simulink model "EKF_04_2014"  (R2015a)
settings: Solver=ode45  StartTime=0.0  StopTime=200  RelTol=1e-3
model workspace: external: MATLAB File Init_Model_02_Simulink.m (data not in the file)
values from neighbouring files (symbols this model uses):
  Cov_nu = [0.005 0 0 0 ... (first row only)    [InitOOSM.m]    (also in InitSIL.m; Init_Model_02_Simulink.m; Init_Model_02_Simulink_SIL1.m)
  Cov_r = [0.003 0 0 ... (first row only)    [InitOOSM.m]    (also in InitSIL.m; Init_Model_02_Simulink.m; Init_Model_02_Simulink_SIL1.m)
  e_force_x = 0    [InitOOSM.m]    (also in InitSIL.m; Init_Model_02_Simulink.m; Init_Model_02_Simulink_SIL1.m)
  e_force_y = 0    [InitOOSM.m]    (also in InitSIL.m; Init_Model_02_Simulink.m; Init_Model_02_Simulink_SIL1.m)
  e_force_z = 0    [InitOOSM.m]    (also in InitSIL.m; Init_Model_02_Simulink.m; Init_Model_02_Simulink_SIL1.m)
  ita = [0.5;0.5;0.5;0.5]    [InitOOSM.m]    (also in InitSIL.m; Init_Model_02_Simulink.m = [0.12; 0.05; -0.15; 0.98]; Init_Model_02_Simulink_SIL1.m)
  n = 0.00    (= 0)    [InitOOSM.m]    (also in InitSIL.m; Init_Model_02_Simulink.m = 0.0012; Init_Model_02_Simulink_SIL1.m)
  P_d = Simulink.Signal    [InitOOSM.m]    (also in InitSIL.m; Init_Model_02_Simulink.m; Init_Model_02_Simulink_SIL1.m)
  P_k = Simulink.Signal    [InitOOSM.m]    (also in InitSIL.m; Init_Model_02_Simulink.m; Init_Model_02_Simulink_SIL1.m)
  p_x = 0.75    [InitOOSM.m]    (also in InitSIL.m; Init_Model_02_Simulink.m; Init_Model_02_Simulink_SIL1.m)
  p_y = 0.125    [InitOOSM.m]    (also in InitSIL.m; Init_Model_02_Simulink.m; Init_Model_02_Simulink_SIL1.m)
  p_z = -0.8    [InitOOSM.m]    (also in InitSIL.m; Init_Model_02_Simulink.m; Init_Model_02_Simulink_SIL1.m)
  parameter_gravitation = 3.986005E+14    (= 398600500000000)    [InitOOSM.m]    (also in InitSIL.m; Init_Model_02_Simulink.m; Init_Model_02_Simulink_SIL1.m)
  rho = [0.04;0;0.3]    [InitOOSM.m]    (also in InitSIL.m; Init_Model_02_Simulink.m = [0.2; 0.1; 0.05]; Init_Model_02_Simulink_SIL1.m)
  rho_c = [-0.00017;   -0.9780;   -0.1854]    [InitOOSM.m]    (also in InitSIL.m = [0.00036;   -0.9865;   -0.1854]; Init_Model_02_Simulink.m = [0; 0; 0.9]; Init_Model_02_Simulink_SIL1.m = [0.00036;   -0.9865;   -0.1854])
  sig_f = 2E-6    (= 2e-06)    [InitOOSM.m]    (also in InitSIL.m; Init_Model_02_Simulink.m; Init_Model_02_Simulink_SIL1.m)
  sig_tau = 2.5E-5    (= 2.5e-05)    [InitOOSM.m]    (also in InitSIL.m; Init_Model_02_Simulink.m; Init_Model_02_Simulink_SIL1.m)
  t_delta = 0.2    [InitOOSM.m]    (also in InitSIL.m; Init_Model_02_Simulink.m = 0.1; Init_Model_02_Simulink_SIL1.m)
  t_Kalman = 0.01    [InitOOSM.m]    (also in InitSIL.m; Init_Model_02_Simulink.m; Init_Model_02_Simulink_SIL1.m)
  t_Sim = 0.001    [InitOOSM.m]    (also in InitSIL.m; Init_Model_02_Simulink.m; Init_Model_02_Simulink_SIL1.m)
  tau_1 = 0    [InitOOSM.m]    (also in InitSIL.m; Init_Model_02_Simulink.m; Init_Model_02_Simulink_SIL1.m)
  tau_2 = 0    [InitOOSM.m]    (also in InitSIL.m; Init_Model_02_Simulink.m; Init_Model_02_Simulink_SIL1.m)
  tau_3 = 0    [InitOOSM.m]    (also in InitSIL.m; Init_Model_02_Simulink.m; Init_Model_02_Simulink_SIL1.m)
  U_n_d = Simulink.Signal    [InitOOSM.m]    (also in InitSIL.m; Init_Model_02_Simulink.m; Init_Model_02_Simulink_SIL1.m)
  W_0 = [1 0 0 0 0 0 ... (first row only)    [InitOOSM.m]    (also in InitSIL.m; Init_Model_02_Simulink.m; Init_Model_02_Simulink_SIL1.m)
  X_a_0 = [0; 0; 0; 1; 0; 0; 0; 0; 0; 0; 0; 0; 0;0;0;0;0;0;0;1]    [InitOOSM.m]    (also in InitSIL.m = [0; 0; 0; 1; 0; 0; 0; 0; 0; 0; 0; 0; 0]; Init_Model_02_Simulink.m = [0; 0; 0; 1; 0; 0; 0; 0; 0; 0; 0; 0; 0]; Init_Model_02_Simulink_SIL1.m = [0;0;0.707;0.707;0.2;-0.02;0.0001;0.02;-1.80;0.50;-0.05;0.00)
  x_d = Simulink.Signal    [InitOOSM.m]    (also in InitSIL.m; Init_Model_02_Simulink.m; Init_Model_02_Simulink_SIL1.m)
  x_k = Simulink.Signal    [InitOOSM.m]    (also in InitSIL.m; Init_Model_02_Simulink.m; Init_Model_02_Simulink_SIL1.m)
undefined symbols (not defined in the file or in its folder): des, gcbh
libraries: simulink x8, dspmtrx3 x2, visionstatistics x1
(part 1 of 5)
settings Model: PauseTimes=0.19  NumberOfSteps=10  SnapshotBufferSize=1  CovSFcnEnable=off  Creator=Iseberg  LastModifiedBy=Ana
settings DebuggingCC: SolverPrmCheckMsg=warning

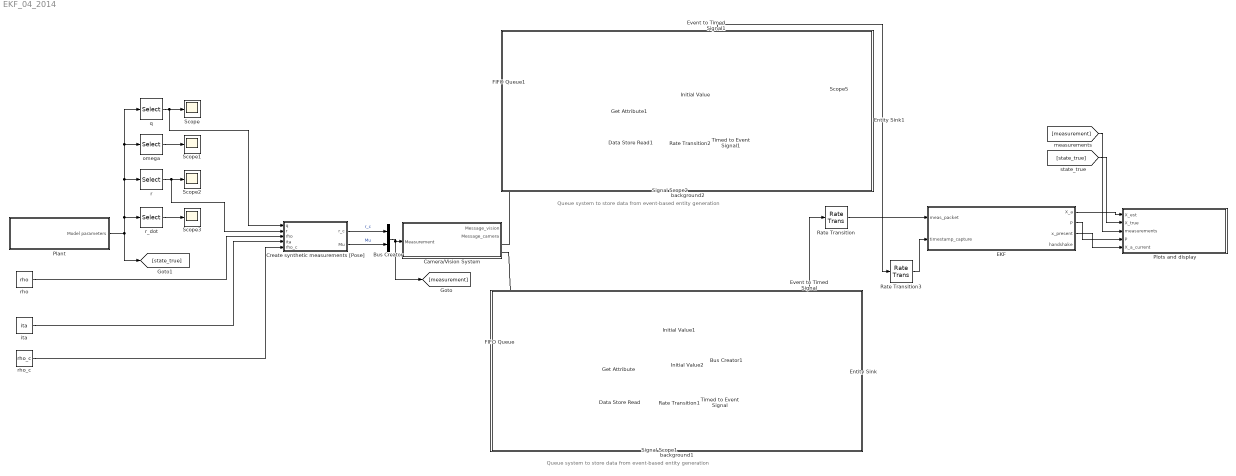
== system EKF_04_2014 ==
  note: Queue system to store data from event-based entity generation
  note: Queue system to store data from event-based entity generation
  Bus Creator : BusCreator  Inputs=2
  Bus Creator1 : BusCreator  Inputs=3
  Camera/Vision System : Subsystem
  Create synthetic measurements [Pose] : Subsystem  TreatAsAtomicUnit=on
  Data Store Read : DataStoreRead  DataStoreName=flag_queue
  Data Store Read1 : DataStoreRead  DataStoreName=flag_queue
  EKF : Subsystem  TreatAsAtomicUnit=on  SystemSampleTime=t_Kalman
  Entity Sink : EntitySink
  Entity Sink1 : EntitySink
  Event to Timed Signal : EventToTimedSignal
  Event to Timed Signal1 : EventToTimedSignal
  FIFO Queue : FIFOQueue  StatNumberInBlock=on
      settings: OutputPortMap=o1
  FIFO Queue1 : FIFOQueue  StatNumberInBlock=on
      settings: OutputPortMap=o1
  Get Attribute : GetAttribute  AttributeName=meas_vector|timestamp_capture|timestamp_processed  AttributeMissing=Error|Error|Error  AttributeDefaultValue=1|1|1  AttributeTreatAsVector=1|1|1  AttributeSendTiming=After entity departure|After entity departure|After entity departure  EvaluatedDefaultAttributeValue={ [];[];[]}
      settings: OutputPortMap=o1,o2,o3
  Get Attribute1 : GetAttribute  AttributeName=timestamp_capture  EvaluatedDefaultAttributeValue={ []}
      settings: OutputPortMap=o1
  Initial Value : InitialValue  InitialValue=-1
  Initial Value1 : InitialValue  InitialValue=-1
  Initial Value2 : InitialValue  InitialValue=-1
  Plant : Subsystem
  Plots and display : Subsystem
  Rate Transition{,1..3} (4 alike) : RateTransition  OutPortSampleTime=t_Kalman
  Scope{,1..3,5} (5 alike) : Scope
      Scope settings: ShowLegends=on  YMin=-1  YMax=1  MaxDataPoints=100000
      Scope1 settings: ShowLegends=on  TimeRange=40
      Scope2 settings: ShowLegends=on  SaveName=ScopeData2
      Scope3 settings: ShowLegends=on  SaveName=ScopeData3
      Scope5 settings: SaveName=ScopeData12
  Signal Scope1 : SignalScope  LoadFcn=des.scope.CallbackSupport('seLoadFcn',gcbh)  StartFcn=des.scope.CallbackSupport('seStartFcn',gcbh)  StopFcn=des.scope.CallbackSupport('seStopFcn',gcbh)
      settings: CopyFcn=des.scope.CallbackSupport('seCopyFcn',gcbh)  DeleteFcn=des.scope.CallbackSupport('seDeleteFcn',gcbh)  PreSaveFcn=des.scope.CallbackSupport('sePreSaveFcn',gcbh)  NameChangeFcn=des.scope.CallbackSupport('seNameChangeFcn',gcbh)  OpenFcn=des.scope.CallbackSupport('seOpenFcn',gcbh)
  Signal Scope2 : SignalScope  LoadFcn=des.scope.CallbackSupport('seLoadFcn',gcbh)  StartFcn=des.scope.CallbackSupport('seStartFcn',gcbh)  StopFcn=des.scope.CallbackSupport('seStopFcn',gcbh)
      settings: CopyFcn=des.scope.CallbackSupport('seCopyFcn',gcbh)  DeleteFcn=des.scope.CallbackSupport('seDeleteFcn',gcbh)  PreSaveFcn=des.scope.CallbackSupport('sePreSaveFcn',gcbh)  NameChangeFcn=des.scope.CallbackSupport('seNameChangeFcn',gcbh)  OpenFcn=des.scope.CallbackSupport('seOpenFcn',gcbh)
  Timed to Event Signal : TimedToEventSignal
  Timed to Event Signal1 : TimedToEventSignal
  background1 : Subsystem
      mask Display: disp('')
  background2 : Subsystem
      mask Display: disp('')
  ita : Constant  Value=ita
  omega : Selector  NumberOfDimensions=2  InputPortWidth=3  IndexOptions=Index vector (dialog),Index vector (dialog)  Indices=[5 6 7],1  OutputSizes=1,1
  q : Selector  NumberOfDimensions=2  InputPortWidth=3  IndexOptions=Index vector (dialog),Index vector (dialog)  Indices=[1 2 3 4],1  OutputSizes=1,1
  r : Selector  NumberOfDimensions=2  InputPortWidth=3  IndexOptions=Index vector (dialog),Index vector (dialog)  Indices=[8 9 10],1  OutputSizes=1,1
  r_dot : Selector  NumberOfDimensions=2  InputPortWidth=3  IndexOptions=Index vector (dialog),Index vector (dialog)  Indices=[11 12 13],1  OutputSizes=1,1
  "rho " : Constant  Value=rho
  rho_c : Constant  Value=rho_c
  wires:
  omega/1 -> Scope1/1
  r_dot/1 -> Scope3/1
  Plant/1(Model parameters) -> [state_true], omega/1, q/1, r/1, r_dot/1
  q/1 -> Create synthetic measurements [Pose]/1(q), Scope/1
  r/1 -> Create synthetic measurements [Pose]/2(r), Scope2/1
  "rho "/1 -> Create synthetic measurements [Pose]/3(rho)
  ita/1 -> Create synthetic measurements [Pose]/4(ita)
  rho_c/1 -> Create synthetic measurements [Pose]/5("rho_c ")
  Create synthetic measurements [Pose]/1(r_c) -> Bus Creator/1  "r_c"
  Create synthetic measurements [Pose]/2(Mu) -> Bus Creator/2  "Mu"
  Bus Creator/1 -> [measurement], Camera/Vision System/1(Measurement)
  Bus Creator1/1 -> Event to Timed Signal/1
  FIFO Queue/1 -> Signal Scope1/1
  Get Attribute/2 -> Initial Value1/1
  Get Attribute/1 -> Bus Creator1/1
  [state_true] -> Plots and display/2(X_true)
  [measurement] -> Plots and display/3(measurements)
  EKF/2(P) -> Plots and display/4(P)
  Event to Timed Signal/1 -> Rate Transition/1
  Data Store Read/1 -> Rate Transition1/1
  Rate Transition1/1 -> Timed to Event Signal/1
  FIFO Queue1/1 -> Signal Scope2/1
  Get Attribute1/1 -> Initial Value/1
  Event to Timed Signal1/1 -> Rate Transition3/1
  Data Store Read1/1 -> Rate Transition2/1
  Rate Transition2/1 -> Timed to Event Signal1/1
  Timed to Event Signal1/1 -> Scope5/1
  Rate Transition3/1 -> EKF/2("timestamp_capture ")
  Rate Transition/1 -> EKF/1(meas_packet)
  Initial Value/1 -> Event to Timed Signal1/1
  Initial Value1/1 -> Bus Creator1/2
  Get Attribute/3 -> Initial Value2/1
  Initial Value2/1 -> Bus Creator1/3
  EKF/1(X_a) -> Plots and display/1(X_est)
  EKF/3(x_present) -> Plots and display/5("X_a_current ")
  connections:
  Camera/Vision System/RConn2 -- FIFO Queue/LConn1
  FIFO Queue/RConn1 -- Get Attribute/LConn1
  Get Attribute/RConn1 -- Entity Sink/LConn1
  Get Attribute1/RConn1 -- Entity Sink1/LConn1
  FIFO Queue1/RConn1 -- Get Attribute1/LConn1
  FIFO Queue1/LConn1 -- Camera/Vision System/RConn1

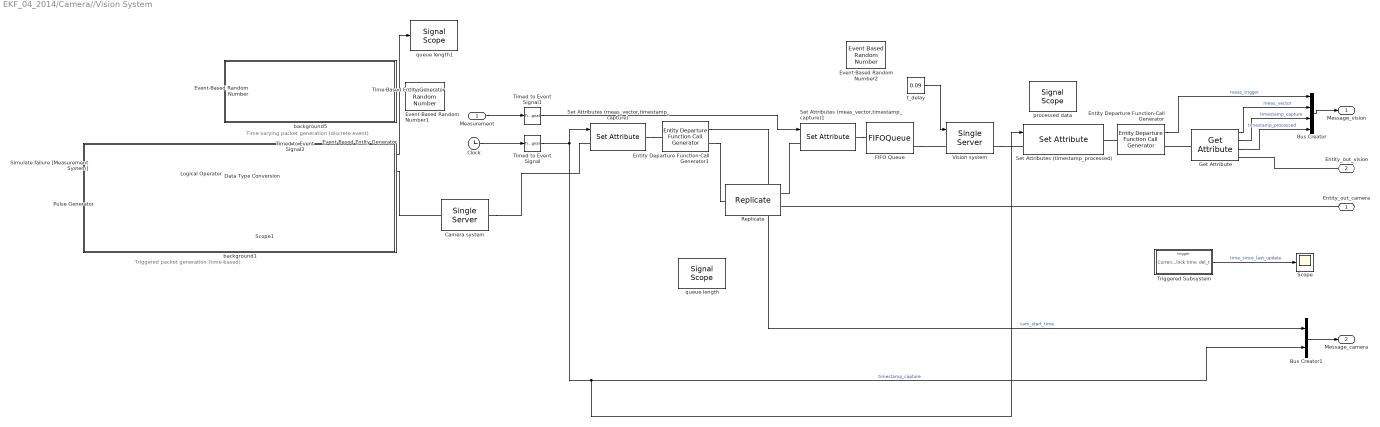
== system EKF_04_2014/Camera//Vision System ==
  note: Triggered packet generation (time-based)
  note: Time-varying packet generation
      | (discrete event)
  Measurement : Inport
  Bus Creator : BusCreator
  Bus Creator1 : BusCreator  Inputs=2
  Camera system : SingleServer  ServiceTime=0
  Clock : Clock
      settings: Decimation=2
  Data Type Conversion : DataTypeConversion
  Entity Departure Function-Call Generator : EntityDepartureFunctionCallGenerator
  Entity Departure Function-Call Generator1 : EntityDepartureFunctionCallGenerator  TimingFunctionCallF1=Before entity departure
  Event-Based Entity Generator : EventBasedEntityGenerator  StatNumberDeparted=on
  Event-Based Random Number : EventBasedRandomNumber  Distribution=Uniform  minUnif=0.09  maxUnif=0.15
  Event-Based Random Number1 : EventBasedRandomNumber  Distribution=Uniform  minUnif=0.08  maxUnif=0.12
  Event-Based Random Number2 : EventBasedRandomNumber  Distribution=Uniform  minUnif=0.08  maxUnif=0.12
  FIFO Queue : FIFOQueue  Capacity=1  StatNumberInBlock=on
      settings: OutputPortMap=o1
  Get Attribute : GetAttribute  AttributeName=meas_vector|timestamp_capture|timestamp_processed  AttributeMissing=Error|Error|Error  AttributeDefaultValue=1|1|1  AttributeTreatAsVector=1|1|1  AttributeSendTiming=After entity departure|After entity departure|After entity departure  EvaluatedDefaultAttributeValue={ [];[];[]}
      settings: OutputPortMap=o1,o2,o3
  Logical Operator : Logic  AllPortsSameDT=off  OutDataTypeStr=boolean
  Pulse Generator : DiscretePulseGenerator  Period=10  SampleTime=t_delta/10
  Replicate : Replicate  NumberOutputPorts=2
  Scope : Scope
  Scope1 : Scope
      settings: SaveName=ScopeData8
  Set Attributes (meas_vector,timestamp_capture) : SetAttribute  AttributeName=timestamp_capture  AttributeFrom=Signal port  EvaluatedAttributeValue={ []}
  Set Attributes (meas_vector,timestamp_capture)1 : SetAttribute  AttributeName=meas_vector  AttributeFrom=Signal port  EvaluatedAttributeValue={ []}
  Set Attributes (timestamp_processed) : SetAttribute  AttributeName=timestamp_processed  AttributeFrom=Signal port  EvaluatedAttributeValue={ []}
  Simulate failure [Measurement System] : Subsystem
  Time-Based Entity Generator : TimeBasedEntityGenerator  Period=t_delta  StatNumberDeparted=on
  Timed to Event Signal : TimedToEventSignal
  Timed to Event Signal1 : TimedToEventSignal
  Timed to Event Signal2 : TimedToEventSignal
  Triggered Subsystem : Subsystem  TreatAsAtomicUnit=on
  Vision system : SingleServer  ServiceTimeFrom=Signal port t  StatNumberDeparted=on
  background1 : Subsystem
      mask Display: disp('')
  background5 : Subsystem
      mask Display: disp('')
  processed data : SignalScope  LoadFcn=des.scope.CallbackSupport('seLoadFcn',gcbh)  StartFcn=des.scope.CallbackSupport('seStartFcn',gcbh)  StopFcn=des.scope.CallbackSupport('seStopFcn',gcbh)
      settings: CopyFcn=des.scope.CallbackSupport('seCopyFcn',gcbh)  DeleteFcn=des.scope.CallbackSupport('seDeleteFcn',gcbh)  PreSaveFcn=des.scope.CallbackSupport('sePreSaveFcn',gcbh)  NameChangeFcn=des.scope.CallbackSupport('seNameChangeFcn',gcbh)  OpenFcn=des.scope.CallbackSupport('seOpenFcn',gcbh)
  queue length : SignalScope  LoadFcn=des.scope.CallbackSupport('seLoadFcn',gcbh)  StartFcn=des.scope.CallbackSupport('seStartFcn',gcbh)  StopFcn=des.scope.CallbackSupport('seStopFcn',gcbh)
      settings: CopyFcn=des.scope.CallbackSupport('seCopyFcn',gcbh)  DeleteFcn=des.scope.CallbackSupport('seDeleteFcn',gcbh)  PreSaveFcn=des.scope.CallbackSupport('sePreSaveFcn',gcbh)  NameChangeFcn=des.scope.CallbackSupport('seNameChangeFcn',gcbh)  OpenFcn=des.scope.CallbackSupport('seOpenFcn',gcbh)
  queue length1 : SignalScope  LoadFcn=des.scope.CallbackSupport('seLoadFcn',gcbh)  StartFcn=des.scope.CallbackSupport('seStartFcn',gcbh)  StopFcn=des.scope.CallbackSupport('seStopFcn',gcbh)
      settings: CopyFcn=des.scope.CallbackSupport('seCopyFcn',gcbh)  DeleteFcn=des.scope.CallbackSupport('seDeleteFcn',gcbh)  PreSaveFcn=des.scope.CallbackSupport('sePreSaveFcn',gcbh)  NameChangeFcn=des.scope.CallbackSupport('seNameChangeFcn',gcbh)  OpenFcn=des.scope.CallbackSupport('seOpenFcn',gcbh)
  t_delay : Constant  Value=0.09
  Entity_out_camera : PMIOPort  Port=1  Side=Right
  Entity_out_vision : PMIOPort  Port=2  Side=Right
  "Message_vision " : Outport
  "Message_camera " : Outport  Port=2
  wires:
  Bus Creator/1 -> "Message_vision "/1
  Timed to Event Signal1/1 -> Set Attributes (meas_vector,timestamp_capture)1/1
  Timed to Event Signal/1 -> Bus Creator1/2, Set Attributes (timestamp_processed)/1, Set Attributes (meas_vector,timestamp_capture)/1  "timestamp_capture"
  Get Attribute/3 -> Bus Creator/4  "timestamp_processed"
  Measurement/1 -> Timed to Event Signal1/1
  Entity Departure Function-Call Generator/1 -> Bus Creator/1  "meas_trigger"
  Get Attribute/2 -> Bus Creator/3  "timestamp_capture"
  Get Attribute/1 -> Bus Creator/2  "meas_vector"
  Clock/1 -> Timed to Event Signal/1
  Triggered Subsystem/1(del_t) -> Scope/1  "time_since_last_update"
  Bus Creator1/1 -> "Message_camera "/1
  t_delay/1 -> Vision system/1
  Entity Departure Function-Call Generator1/1 -> Bus Creator1/1  "cam_start_time"
  Simulate failure [Measurement System]/1(Out1) -> Logical Operator/1
  Logical Operator/1 -> Scope1/1, Data Type Conversion/1
  Data Type Conversion/1 -> Timed to Event Signal2/1
  Timed to Event Signal2/1 -> Event-Based Entity Generator/1
  Event-Based Random Number/1 -> ?
  Pulse Generator/1 -> Logical Operator/2
  Event-Based Entity Generator/1 -> queue length1/1
  connections:
  Entity Departure Function-Call Generator/LConn1 -- Set Attributes (timestamp_processed)/RConn1
  Vision system/RConn1 -- Set Attributes (timestamp_processed)/LConn1
  Get Attribute/LConn1 -- Entity Departure Function-Call Generator/RConn1
  Camera system/RConn1 -- Set Attributes (meas_vector,timestamp_capture)/LConn1
  Entity Departure Function-Call Generator1/RConn1 -- Replicate/LConn1
  Set Attributes (meas_vector,timestamp_capture)/RConn1 -- Entity Departure Function-Call Generator1/LConn1
  FIFO Queue/RConn1 -- Vision system/LConn1
  Entity_out_vision/RConn1 -- Get Attribute/RConn1
  Event-Based Entity Generator/RConn1 -- Camera system/LConn1
  Replicate/RConn1 -- Set Attributes (meas_vector,timestamp_capture)1/LConn1
  Entity_out_camera/RConn1 -- Replicate/RConn2
  Set Attributes (meas_vector,timestamp_capture)1/RConn1 -- FIFO Queue/LConn1

== system EKF_04_2014/Create synthetic measurements [Pose] ==
  q : Inport
  r : Inport  Port=2
  rho : Inport  Port=3
  ita : Inport  Port=4
  "rho_c " : Inport  Port=5
  "Create Measurements [Orientation] " : Subsystem
  Create Measurements [Position] : Subsystem
  r_c : Outport
  Mu : Outport  Port=2
  wires:
  "rho_c "/1 -> Create Measurements [Position]/4("rho_c ")
  rho/1 -> Create Measurements [Position]/3(rho)
  Create Measurements [Position]/1(r_c) -> r_c/1
  ita/1 -> "Create Measurements [Orientation] "/2("ita ")
  "Create Measurements [Orientation] "/1(Mu) -> Mu/1
  r/1 -> Create Measurements [Position]/1(r)
  q/1 -> Create Measurements [Position]/2(q), "Create Measurements [Orientation] "/1(q)

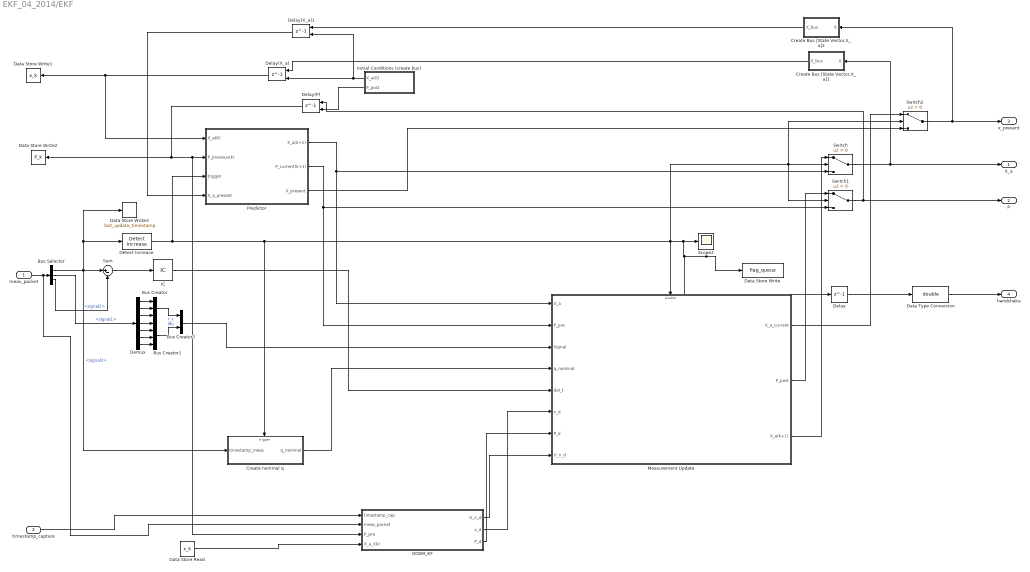
== system EKF_04_2014/EKF ==
  meas_packet : Inport
  "timestamp_capture " : Inport  Port=2
  Bus Creator : BusCreator  Inputs=3
  Bus Creator1 : BusCreator
  Bus Creator2 : BusCreator  Inputs=2
  Bus Selector : BusSelector  OutputSignals=signal3,signal1,signal2
  Create Bus [State Vector,X_a]1 : Subsystem
  Create Bus [State Vector,X_a]2 : Subsystem
  Create nominal q : Subsystem  TreatAsAtomicUnit=on
  Data Store Read : DataStoreRead  DataStoreName=x_k
  Data Store Write : DataStoreWrite  DataStoreName=flag_queue
  Data Store Write1 : DataStoreWrite  DataStoreName=x_k
  Data Store Write2 : DataStoreWrite  DataStoreName=P_k
  Data Store Write3 : DataStoreWrite  DataStoreName=last_update_timestamp
  Data Type Conversion : DataTypeConversion  OutDataTypeStr=double  LockScale=on
  Delay : Delay  DelayLength=1  InitialCondition=0
  Delay(P) : Delay  DelayLength=1  InitialConditionSource=Input port  InitialCondition=0  SampleTime=t_Kalman
      settings: InputPortMap=u0,p4
  Delay(X_a) : Delay  DelayLength=1  InitialConditionSource=Input port  InitialCondition=0  SampleTime=t_Kalman
      settings: InputPortMap=u0,p4
  Delay(X_a)1 : Delay  DelayLength=1  InitialConditionSource=Input port  InitialCondition=0  SampleTime=t_Kalman
      settings: InputPortMap=u0,p4
  Demux : Demux  Outputs=7
  Detect Increase : simulink/Logic and Bit Operations/Detect Increase  vinit=-1  InputProcessing=Inherited  OutDataTypeStr=boolean
  IC : InitialCondition  Value=0
  Initial Conditions (create bus) : Subsystem
  Measurement Update : Subsystem  TreatAsAtomicUnit=on
  OOSM_KF : Subsystem  TreatAsAtomicUnit=on  SystemSampleTime=t_Kalman
  Predictor : Subsystem  TreatAsAtomicUnit=on  SystemSampleTime=t_Kalman
  Scope2 : Scope
      settings: YMin=0  YMax=1  SaveName=ScopeData5
  Sum : Sum  Inputs=|+-
  Switch : Switch  Criteria=u2 > Threshold
  Switch1 : Switch  Criteria=u2 > Threshold
  Switch2 : Switch  Criteria=u2 > Threshold
  X_a : Outport
  P : Outport  Port=2
  x_present : Outport  Port=3
  handshake : Outport  Port=4
  wires:
  meas_packet/1 -> OOSM_KF/2("meas_packet "), Bus Selector/1
  Bus Selector/2 -> Demux/1  "<signal1>"
  Bus Selector/1 -> Sum/1, Detect Increase/1, Data Store Write3/1, Create nominal q/1(timestamp_meas)  "<signal3>"
  Predictor/2(P_current(k+1)) -> Switch1/3, Measurement Update/2(P_pre)
  Measurement Update/3(X_a(k+1)) -> Switch/1
  Measurement Update/2(P_post) -> Switch1/1
  Switch/1 -> Create Bus [State Vector,X_a]1/1(X), X_a/1
  Initial Conditions (create bus)/2("P_post ") -> Delay(P)/2
  Switch1/1 -> Delay(P)/1, P/1
  Delay(P)/1 -> OOSM_KF/3(P_pre), Predictor/2(P_previous(k)), Data Store Write2/1
  Demux/1 -> Bus Creator/1
  Demux/2 -> Bus Creator/2
  Demux/3 -> Bus Creator/3
  Demux/4 -> Bus Creator1/1
  Demux/5 -> Bus Creator1/2
  Demux/6 -> Bus Creator1/3
  Demux/7 -> Bus Creator1/4
  Bus Creator/1 -> Bus Creator2/1  "r_c"
  Bus Creator1/1 -> Bus Creator2/2  "Mu"
  Create Bus [State Vector,X_a]1/1(X_bus) -> Delay(X_a)/1
  Predictor/1(X_a(k+1)) -> Measurement Update/1(X_a), Switch/3
  Initial Conditions (create bus)/1("X_a(0) ") -> Delay(X_a)1/2, Delay(X_a)/2
  Create nominal q/1(q_nominal) -> Measurement Update/4("q_nominal ")
  Bus Creator2/1 -> Measurement Update/3(Signal)
  Detect Increase/1 -> Predictor/3(trigger), Measurement Update/Enable, Switch2/2, Switch1/2, Switch/2, Delay/1, Data Store Write/1, Scope2/1, Create nominal q/Trigger
  Predictor/3(X_present) -> Switch2/3
  Bus Selector/3 -> Sum/2  "<signal2>"
  Sum/1 -> IC/1
  IC/1 -> Measurement Update/5(del_t)
  Delay(X_a)1/1 -> Predictor/4(X_a_present)
  Measurement Update/1(X_a_current) -> Switch2/1
  Create Bus [State Vector,X_a]2/1(X_bus) -> Delay(X_a)1/1
  Switch2/1 -> Create Bus [State Vector,X_a]2/1(X), x_present/1
  Delay/1 -> Data Type Conversion/1
  Data Type Conversion/1 -> handshake/1
  "timestamp_capture "/1 -> OOSM_KF/1("timestamp_cap ")
  OOSM_KF/1(U_n_d) -> Measurement Update/8(U_n_d)
  OOSM_KF/2(x_d) -> Measurement Update/6(x_d)
  OOSM_KF/3(P_d) -> Measurement Update/7(P_d)
  Delay(X_a)/1 -> Predictor/1(X_a(K)), Data Store Write1/1
  Data Store Read/1 -> OOSM_KF/4(X_a_\(k))

== system EKF_04_2014/Plant ==
  Dynamic Model (Differential equations) : Subsystem
  Initial Conditions (create bus) : Subsystem
  Integrator : Integrator  InitialConditionSource=external
  Selector2 : Selector  NumberOfDimensions=2  InputPortWidth=3  IndexOptions=Index vector (dialog),Index vector (dialog)  Indices=[1:13],1  OutputSizes=1,1
  Model parameters : Outport
  wires:
  Integrator/1 -> Model parameters/1, Dynamic Model (Differential equations)/1(X_a(t))
  Initial Conditions (create bus)/1("X_a(0) ") -> Selector2/1
  Selector2/1 -> Integrator/2
  Dynamic Model (Differential equations)/1(X_a(t+1)) -> Integrator/1

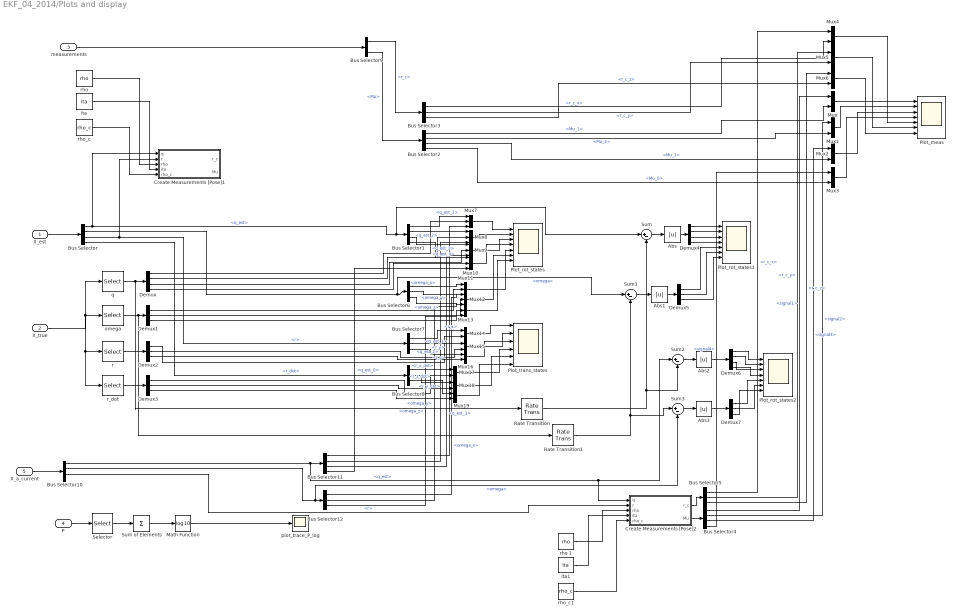
== system EKF_04_2014/Plots and display ==
  X_est : Inport
  X_true : Inport  Port=2
  measurements : Inport  Port=3
  P : Inport  Port=4
  "X_a_current " : Inport  Port=5
  Abs{,1..3} (4 alike) : Abs
  Bus Selector : BusSelector  OutputSignals=q_est,omega,r,r_dot
  Bus Selector1 : BusSelector  OutputSignals=q_est_1,q_est_2,q_est_3,q_est_0
  Bus Selector10 : BusSelector  OutputSignals=q_est,omega,r,r_dot
  Bus Selector11 : BusSelector  OutputSignals=q_est_1,q_est_2,q_est_3,q_est_0
  Bus Selector12 : BusSelector  OutputSignals=omega_x,omega_y,omega_z
  Bus Selector2 : BusSelector  OutputSignals=Mu_1,Mu_2,Mu_3,Mu_0
  Bus Selector3 : BusSelector  OutputSignals=r_c_x,r_c_y,r_c_z
  Bus Selector4 : BusSelector  OutputSignals=signal1,signal2,signal3,signal4
  Bus Selector5 : BusSelector  OutputSignals=r_c_x,r_c_y,r_c_z
  Bus Selector6 : BusSelector  OutputSignals=omega_x,omega_y,omega_z
  Bus Selector7 : BusSelector  OutputSignals=r_x,r_y,r_z
  Bus Selector8 : BusSelector  OutputSignals=r_x_dot,r_y_dot,r_z_dot
  Bus Selector9 : BusSelector  OutputSignals=r_c,Mu
  Create Measurements [Pose]1 : Subsystem
  Create Measurements [Pose]2 : Subsystem
  Demux : Demux
  Demux{1..3,5,7} (5 alike) : Demux  Outputs=3
  Demux4 : Demux
  Demux6 : Demux
  Math Function : Math  Operator=log10  SaturateOnIntegerOverflow=on
  Mux{,1..6,14..19} (13 alike) : Mux  Inputs=2
  Mux{7..13} (7 alike) : Mux  Inputs=3
  "Plot_meas " : Scope  NumInputPorts=7
      settings: ShowLegends=on  TimeRange=200  YMin=-1~-5~-5~-5~-5~-5~-5  YMax=1~5~5~5~5~5~5  SaveName=ScopeData9
  Plot_rot_states : Scope  NumInputPorts=7
      settings: ShowLegends=on  TimeRange=100  YMin=-0.5~-1~-1~-1~-0.2~-0.3~-0.75  YMax=0.6~1~1~1~0.9~0.4~0.75  SaveName=ScopeData24
  Plot_rot_states1 : Scope  NumInputPorts=7
      settings: ShowLegends=on  TimeRange=100  YMin=-1~-1~-1~-0.75~0~-0.4~-1  YMax=1~1~1~1~1~0.4~1  SaveName=ScopeData14
  Plot_rot_states2 : Scope  NumInputPorts=7
      settings: ShowLegends=on  TimeRange=100  YMin=-3.46945e-18~-3.46945e-18~-1.38778e-17~-2.77556e-17~0.05~1.38778e-17~5.55112e-17  YMax=0.1~0.14~0.175~0.35~0.35~0.25~0.9  SaveName=ScopeData15
  "Plot_trans_states " : Scope  NumInputPorts=6
      settings: ShowLegends=on  TimeRange=100  YMin=-0.5~0~-1~-0.05~-0.025~-0.15  YMax=3~1.25~0~0.4~0.15~0.025  SaveName=ScopeData11
  Rate Transition : RateTransition
  Rate Transition1 : RateTransition
  Selector : Selector  NumberOfDimensions=2  InputPortWidth=3  IndexOptions=Index vector (dialog),Index vector (dialog)  Indices=[1:12],[1:12]  OutputSizes=1,1
  Sum{,1..3} (4 alike) : Sum  Inputs=|+-
  Sum of Elements : Sum  Inputs=+
  ita : Constant  Value=ita
  ita1 : Constant  Value=ita
  omega : Selector  NumberOfDimensions=2  InputPortWidth=3  IndexOptions=Index vector (dialog),Index vector (dialog)  Indices=[5 6 7],1  OutputSizes=1,1
  plot_trace_P_log : Scope
      settings: ShowLegends=on  TimeRange=120  YMin=-2.637825272860399  YMax=-2.50866879562702  SaveName=ScopeData4
  q : Selector  NumberOfDimensions=2  InputPortWidth=3  IndexOptions=Index vector (dialog),Index vector (dialog)  Indices=[1 2 3 4],1  OutputSizes=1,1
  r : Selector  NumberOfDimensions=2  InputPortWidth=3  IndexOptions=Index vector (dialog),Index vector (dialog)  Indices=[8 9 10],1  OutputSizes=1,1
  r_dot : Selector  NumberOfDimensions=2  InputPortWidth=3  IndexOptions=Index vector (dialog),Index vector (dialog)  Indices=[11 12 13],1  OutputSizes=1,1
  "rho " : Constant  Value=rho
  rho 1 : Constant  Value=rho
  rho_c : Constant  Value=rho_c
  rho_c1 : Constant  Value=rho_c
  wires:
  Bus Selector/1 -> Create Measurements [Pose]1/1(q), Sum/1, Bus Selector1/1  "<q_est>"
  Bus Selector/3 -> Create Measurements [Pose]1/2(r), Bus Selector7/1  "<r>"
  Bus Selector1/1 -> Mux7/1  "<q_est_1>"
  Mux7/1 -> Plot_rot_states/1
  Demux/1 -> Mux7/2
  Bus Selector1/2 -> Mux8/1  "<q_est_2>"
  Demux/2 -> Mux8/2
  Bus Selector1/3 -> Mux9/1  "<q_est_3>"
  Demux/3 -> Mux9/2
  Bus Selector1/4 -> Mux10/1  "<q_est_0>"
  Demux/4 -> Mux10/2
  Mux8/1 -> Plot_rot_states/2
  Mux9/1 -> Plot_rot_states/3
  Mux10/1 -> Plot_rot_states/4
  Bus Selector/2 -> Sum1/1, Bus Selector6/1  "<omega>"
  Bus Selector6/1 -> Mux11/1  "<omega_x>"
  Demux1/1 -> Mux11/2
  Bus Selector6/2 -> Mux12/1  "<omega_y>"
  Demux1/2 -> Mux12/2
  Bus Selector6/3 -> Mux13/1  "<omega_z>"
  Demux1/3 -> Mux13/2
  Mux11/1 -> Plot_rot_states/5
  Mux12/1 -> Plot_rot_states/6
  Mux13/1 -> Plot_rot_states/7
  Bus Selector7/1 -> Mux14/1  "<r_x>"
  Demux2/1 -> Mux14/2
  Bus Selector7/2 -> Mux15/1  "<r_y>"
  Demux2/2 -> Mux15/2
  Bus Selector7/3 -> Mux16/1  "<r_z>"
  Demux2/3 -> Mux16/2
  Mux14/1 -> "Plot_trans_states "/1
  Mux15/1 -> "Plot_trans_states "/2
  Mux16/1 -> "Plot_trans_states "/3
  Bus Selector/4 -> Bus Selector8/1  "<r_dot>"
  Bus Selector8/1 -> Mux17/1  "<r_x_dot>"
  Demux3/1 -> Mux17/2
  Bus Selector8/2 -> Mux18/1  "<r_y_dot>"
  Demux3/2 -> Mux18/2
  Bus Selector8/3 -> Mux19/1  "<r_z_dot>"
  Demux3/3 -> Mux19/2
  Mux17/1 -> "Plot_trans_states "/4
  Mux18/1 -> "Plot_trans_states "/5
  Mux19/1 -> "Plot_trans_states "/6
  X_est/1 -> Bus Selector/1
  X_true/1 -> r_dot/1, r/1, omega/1, q/1
  q/1 -> Rate Transition/1, Demux/1
  omega/1 -> Rate Transition1/1, Demux1/1
  r_dot/1 -> Demux3/1
  r/1 -> Demux2/1
  Bus Selector2/1 -> Mux/2  "<Mu_1>"
  Bus Selector2/2 -> Mux1/2  "<Mu_2>"
  Bus Selector2/3 -> Mux2/2  "<Mu_3>"
  Bus Selector4/4 -> Mux3/1  "<signal4>"
  Bus Selector2/4 -> Mux3/2  "<Mu_0>"
  Mux/1 -> "Plot_meas "/1
  Mux1/1 -> "Plot_meas "/2
  Mux2/1 -> "Plot_meas "/3
  Mux3/1 -> "Plot_meas "/4
  Bus Selector3/1 -> Mux4/2  "<r_c_x>"
  Bus Selector3/2 -> Mux5/2  "<r_c_y>"
  Bus Selector3/3 -> Mux6/2  "<r_c_z>"
  Mux4/1 -> "Plot_meas "/5
  Mux5/1 -> "Plot_meas "/6
  Mux6/1 -> "Plot_meas "/7
  "rho "/1 -> Create Measurements [Pose]1/3(rho)
  ita/1 -> Create Measurements [Pose]1/4(ita)
  rho_c/1 -> Create Measurements [Pose]1/5("rho_c ")
  measurements/1 -> Bus Selector9/1
  Bus Selector9/1 -> Bus Selector3/1  "<r_c>"
  Bus Selector9/2 -> Bus Selector2/1  "<Mu>"
  P/1 -> Selector/1
  Selector/1 -> Sum of Elements/1
  Sum of Elements/1 -> Math Function/1
  Math Function/1 -> plot_trace_P_log/1
  "X_a_current "/1 -> Bus Selector10/1
  Bus Selector10/1 -> Create Measurements [Pose]2/1(q), Sum2/1, Bus Selector11/1  "<q_est>"
  Bus Selector10/2 -> Sum3/2, Bus Selector12/1  "<omega>"
  Rate Transition/1 -> Sum2/2, Sum/2
  Sum/1 -> Abs/1
  Abs/1 -> Demux4/1
  Demux4/1 -> Plot_rot_states1/1
  Demux4/2 -> Plot_rot_states1/2
  Demux4/3 -> Plot_rot_states1/3
  Demux4/4 -> Plot_rot_states1/4
  Rate Transition1/1 -> Sum3/1, Sum1/2
  Sum1/1 -> Abs1/1
  Demux5/1 -> Plot_rot_states1/5
  Demux5/2 -> Plot_rot_states1/6
  Demux5/3 -> Plot_rot_states1/7
  Abs1/1 -> Demux5/1
  Sum2/1 -> Abs2/1
  Sum3/1 -> Abs3/1
  Abs2/1 -> Demux6/1
  Demux6/1 -> Plot_rot_states2/1
  Demux6/2 -> Plot_rot_states2/2
  Demux6/3 -> Plot_rot_states2/3
  Demux6/4 -> Plot_rot_states2/4
  Abs3/1 -> Demux7/1
  Demux7/1 -> Plot_rot_states2/5
  Demux7/2 -> Plot_rot_states2/6
  Demux7/3 -> Plot_rot_states2/7
  Bus Selector11/4 -> Mux10/3  "<q_est_0>"
  Bus Selector11/1 -> Mux7/3  "<q_est_1>"
  Bus Selector11/2 -> Mux8/3  "<q_est_2>"
  Bus Selector11/3 -> Mux9/3  "<q_est_3>"
  Bus Selector12/1 -> Mux11/3  "<omega_x>"
  Bus Selector12/2 -> Mux12/3  "<omega_y>"
  Bus Selector12/3 -> Mux13/3  "<omega_z>"
  Bus Selector10/3 -> Create Measurements [Pose]2/2(r)  "<r>"
  rho 1/1 -> Create Measurements [Pose]2/3(rho)
  ita1/1 -> Create Measurements [Pose]2/4(ita)
  rho_c1/1 -> Create Measurements [Pose]2/5("rho_c ")
  Create Measurements [Pose]2/2(Mu) -> Bus Selector4/1
  Bus Selector4/3 -> Mux2/1  "<signal3>"
  Bus Selector4/2 -> Mux1/1  "<signal2>"
  Bus Selector4/1 -> Mux/1  "<signal1>"
  Create Measurements [Pose]2/1(r_c) -> Bus Selector5/1
  Bus Selector5/1 -> Mux4/1  "<r_c_x>"
  Bus Selector5/2 -> Mux5/1  "<r_c_y>"
  Bus Selector5/3 -> Mux6/1  "<r_c_z>"

== system EKF_04_2014/background1 ==

== system EKF_04_2014/background2 ==

== system EKF_04_2014/Camera//Vision System/Simulate failure [Measurement System] ==
  Add : Sum  Inputs=+++
  Step : Step  Time=0  SampleTime=t_Sim
  Step1 : Step  Time=50  After=-1  SampleTime=t_Sim
  Step2 : Step  Time=60  After=8  SampleTime=t_Sim
  Out1 : Outport
  wires:
  Add/1 -> Out1/1
  Step/1 -> Add/2

== system EKF_04_2014/Camera//Vision System/Triggered Subsystem ==
  Current Clock time : Inport
  Trigger : TriggerPort  TriggerType=function-call
  Delay : Delay  DelayLength=1  InitialCondition=0
  Sum : Sum  Inputs=|+-
  del_t : Outport
  wires:
  Current Clock time/1 -> Sum/1, Delay/1
  Sum/1 -> del_t/1
  Delay/1 -> Sum/2

== system EKF_04_2014/Camera//Vision System/background1 ==

== system EKF_04_2014/Camera//Vision System/background5 ==

== system EKF_04_2014/Create synthetic measurements [Pose]/Create Measurements [Orientation]  ==
  q : Inport
  "ita " : Inport  Port=2
  Bus Creator : BusCreator
  Demux : Demux
  Demux1 : Demux
  MATLAB Function : MATLAB Function  TreatAsAtomicUnit=on
  Mux : Mux
  Product : Product  Multiplication=Matrix(*)
  Quaternion norm : Subsystem
  Selector : Selector  NumberOfDimensions=2  InputPortWidth=3  IndexOptions=Index vector (dialog),Index vector (dialog)  Indices=[4 1 2 3],1  OutputSizes=1,1
  Selector1 : Selector  NumberOfDimensions=2  InputPortWidth=3  IndexOptions=Index vector (dialog),Index vector (dialog)  Indices=[2 3 4 1],1  OutputSizes=1,1
  "flag " : Constant  Value=0
  Mu : Outport
  wires:
  Selector/1 -> Quaternion norm/1(q)
  "flag "/1 -> MATLAB Function/2(flag)
  MATLAB Function/1(CrossTensor) -> Product/1
  "ita "/1 -> MATLAB Function/1(q)
  Quaternion norm/1(normalized_q) -> Selector1/1
  Mux/1 -> Selector/1
  Demux1/4 -> Bus Creator/4  "Mu_0"
  Selector1/1 -> Demux1/1  "Mu"
  Demux1/1 -> Bus Creator/1  "Mu_1"
  Demux1/2 -> Bus Creator/2  "Mu_2"
  Demux1/3 -> Bus Creator/3  "Mu_3"
  Bus Creator/1 -> Mu/1  "Mu"
  q/1 -> Product/2
  Product/1 -> Demux/1
  Demux/1 -> Mux/1
  Demux/2 -> Mux/2
  Demux/3 -> Mux/3
  Demux/4 -> Mux/4

== system EKF_04_2014/Create synthetic measurements [Pose]/Create Measurements [Position] ==
  r : Inport
  q : Inport  Port=2
  rho : Inport  Port=3
  "rho_c " : Inport  Port=4
  Add : Sum  Inputs=+++
  Bus Creator : BusCreator  Inputs=3
  "Create Rotation Matrix " : Subsystem
  Demux : Demux  Outputs=3
  Product : Product  Multiplication=Matrix(*)
  r_c : Outport
  wires:
  Product/1 -> Add/3
  "Create Rotation Matrix "/1(R) -> Product/1
  Demux/1 -> Bus Creator/1  "r_c_x"
  rho/1 -> Product/2
  "rho_c "/1 -> Add/1
  q/1 -> "Create Rotation Matrix "/1(q)
  Bus Creator/1 -> r_c/1  "r_c"
  r/1 -> Add/2
  Add/1 -> Demux/1
  Demux/2 -> Bus Creator/2  "r_c_y"
  Demux/3 -> Bus Creator/3  "r_c_z"

== system EKF_04_2014/EKF/Create Bus [State Vector,X_a]1 ==
  X : Inport
  Bus Creator2 : BusCreator
  Bus Creator3 : BusCreator  Inputs=3
  Bus Creator4 : BusCreator  Inputs=3
  Bus Creator5 : BusCreator  Inputs=3
  Bus Creator6 : BusCreator
  Demux1 : Demux  Outputs=13
  X_bus : Outport
  wires:
  Demux1/13 -> Bus Creator5/3  "r_z_dot"
  Demux1/12 -> Bus Creator5/2  "r_y_dot"
  Demux1/11 -> Bus Creator5/1  "r_x_dot"
  Demux1/10 -> Bus Creator4/3  "r_z"
  Demux1/9 -> Bus Creator4/2  "r_y"
  Demux1/8 -> Bus Creator4/1  "r_x"
  Demux1/7 -> Bus Creator3/3  "omega_z"
  Demux1/6 -> Bus Creator3/2  "omega_y"
  Demux1/5 -> Bus Creator3/1  "omega_x"
  Demux1/4 -> Bus Creator2/4  "q_est_0"
  Demux1/3 -> Bus Creator2/3  "q_est_3"
  Demux1/2 -> Bus Creator2/2  "q_est_2"
  Demux1/1 -> Bus Creator2/1  "q_est_1"
  X/1 -> Demux1/1
  Bus Creator6/1 -> X_bus/1
  Bus Creator5/1 -> Bus Creator6/4  "r_dot"
  Bus Creator4/1 -> Bus Creator6/3  "r"
  Bus Creator3/1 -> Bus Creator6/2  "omega"
  Bus Creator2/1 -> Bus Creator6/1  "q_est"

== system EKF_04_2014/EKF/Create Bus [State Vector,X_a]2 ==
  X : Inport
  Bus Creator2 : BusCreator
  Bus Creator3 : BusCreator  Inputs=3
  Bus Creator4 : BusCreator  Inputs=3
  Bus Creator5 : BusCreator  Inputs=3
  Bus Creator6 : BusCreator
  Demux1 : Demux  Outputs=13
  X_bus : Outport
  wires:
  Bus Creator2/1 -> Bus Creator6/1  "q_est"
  Bus Creator3/1 -> Bus Creator6/2  "omega"
  Bus Creator4/1 -> Bus Creator6/3  "r"
  Bus Creator5/1 -> Bus Creator6/4  "r_dot"
  Bus Creator6/1 -> X_bus/1
  X/1 -> Demux1/1
  Demux1/1 -> Bus Creator2/1  "q_est_1"
  Demux1/2 -> Bus Creator2/2  "q_est_2"
  Demux1/3 -> Bus Creator2/3  "q_est_3"
  Demux1/4 -> Bus Creator2/4  "q_est_0"
  Demux1/5 -> Bus Creator3/1  "omega_x"
  Demux1/6 -> Bus Creator3/2  "omega_y"
  Demux1/7 -> Bus Creator3/3  "omega_z"
  Demux1/8 -> Bus Creator4/1  "r_x"
  Demux1/9 -> Bus Creator4/2  "r_y"
  Demux1/10 -> Bus Creator4/3  "r_z"
  Demux1/11 -> Bus Creator5/1  "r_x_dot"
  Demux1/12 -> Bus Creator5/2  "r_y_dot"
  Demux1/13 -> Bus Creator5/3  "r_z_dot"

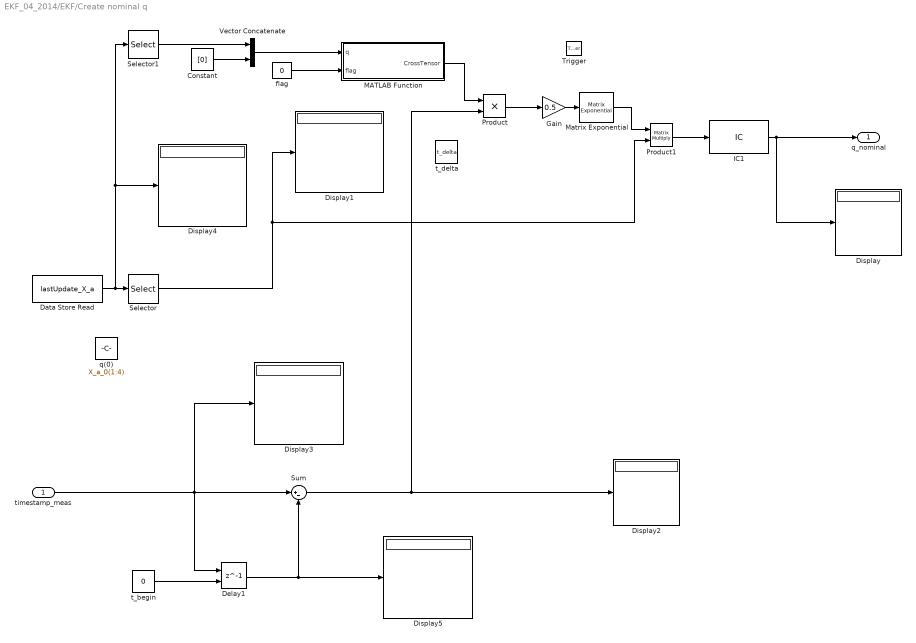
== system EKF_04_2014/EKF/Create nominal q ==
  timestamp_meas : Inport
  Trigger : TriggerPort  PortDimensions=1
  Constant : Constant  Value=[0]
  Data Store Read : DataStoreRead  DialogController=Simulink.DDGSource  DataStoreName=lastUpdate_X_a  DataStoreElements=lastUpdate_X_a
  Delay1 : Delay  DelayLength=1  InitialConditionSource=Input port  InitialCondition=0
      settings: InputPortMap=u0,p4
  Display{,1..5} (6 alike) : Display
  Gain : Gain  Gain=0.5
  IC1 : InitialCondition  Value=X_a_0(1:4)
  MATLAB Function : MATLAB Function  TreatAsAtomicUnit=on
  Matrix Exponential : dspmtrx3/Matrix Exponential
  Product : Product
  Product1 : Product  Multiplication=Matrix(*)
  Selector : Selector  InputPortWidth=13  Indices=[1:4]
  Selector1 : Selector  InputPortWidth=13  Indices=[5:7]
  Sum : Sum  Inputs=|+-
  Vector Concatenate : Concatenate
  flag : Constant  Value=0
  q(0) : Constant  Value=X_a_0(1:4)
  t_begin : Constant  Value=0
  "t_delta " : Constant  Value=t_delta
  q_nominal : Outport
  wires:
  MATLAB Function/1(CrossTensor) -> Product/1
  Sum/1 -> Display2/1, Product/2
  Selector1/1 -> Vector Concatenate/1
  Constant/1 -> Vector Concatenate/2
  flag/1 -> MATLAB Function/2(flag)
  Product/1 -> Gain/1
  Vector Concatenate/1 -> MATLAB Function/1(q)
  Product1/1 -> IC1/1
  Gain/1 -> Matrix Exponential/1
  Matrix Exponential/1 -> Product1/1
  IC1/1 -> Display/1, q_nominal/1
  Selector/1 -> Product1/2, Display1/1
  Data Store Read/1 -> Display4/1, Selector1/1, Selector/1
  timestamp_meas/1 -> Display3/1, Delay1/1, Sum/1
  Delay1/1 -> Display5/1, Sum/2
  t_begin/1 -> Delay1/2

== system EKF_04_2014/EKF/Initial Conditions (create bus) ==
  Bus Creator : BusCreator
  Bus Creator1 : BusCreator  Inputs=3
  Bus Creator2 : BusCreator  Inputs=3
  Bus Creator3 : BusCreator  Inputs=3
  Bus Creator4 : BusCreator  NonVirtualBus=on
  Demux : Demux  Outputs=13
  Initial conditions (null vector) : Constant  Value=[X_a_0]
  Initial conditions (known) : FromFile  FileName=X_a_0_Model_02.mat
  P_post : Constant  Value=0.1*eye(12,12)  VectorParams1D=off
  "X_a(0) " : Outport
  "P_post " : Outport  Port=2
  wires:
  Demux/1 -> Bus Creator/1  "q_1"
  Demux/2 -> Bus Creator/2  "q_2"
  Demux/3 -> Bus Creator/3  "q_3"
  Demux/4 -> Bus Creator/4  "q_0"
  Demux/5 -> Bus Creator1/1  "omega_x"
  Demux/6 -> Bus Creator1/2  "omega_y"
  Demux/7 -> Bus Creator1/3  "omega_z"
  Demux/8 -> Bus Creator2/1  "r_x"
  Demux/9 -> Bus Creator2/2  "r_y"
  Demux/10 -> Bus Creator2/3  "r_z"
  Demux/11 -> Bus Creator3/1  "r_x_dot"
  Demux/12 -> Bus Creator3/2  "r_y_dot"
  Demux/13 -> Bus Creator3/3  "r_z_dot"
  Bus Creator/1 -> Bus Creator4/1  "q_est"
  Bus Creator1/1 -> Bus Creator4/2  "omega"
  Bus Creator2/1 -> Bus Creator4/3  "r"
  Bus Creator3/1 -> Bus Creator4/4  "r_dot"
  Bus Creator4/1 -> "X_a(0) "/1  "X_a(0)"
  P_post/1 -> "P_post "/1
  Initial conditions (null vector)/1 -> Demux/1

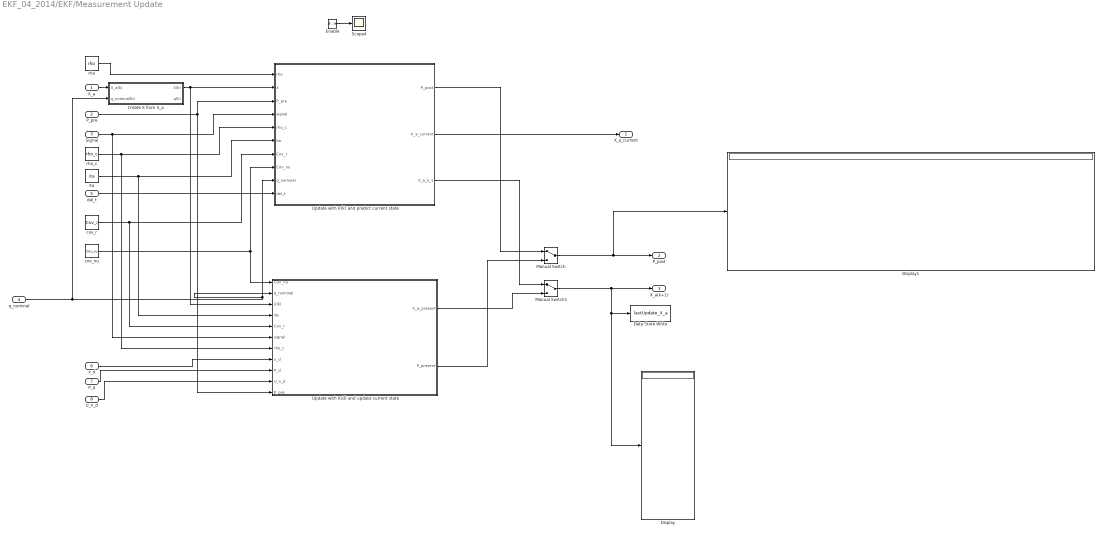
== system EKF_04_2014/EKF/Measurement Update ==
  X_a : Inport
  P_pre : Inport  Port=2
  Signal : Inport  Port=3
  "q_nominal " : Inport  Port=4
  del_t : Inport  Port=5
  x_d : Inport  Port=6
  P_d : Inport  Port=7
  U_n_d : Inport  Port=8
  Enable : EnablePort  ShowOutputPort=on
  Create X from X_a : Subsystem
  Data Store Write : DataStoreWrite  DialogController=Simulink.DDGSource  DataStoreName=lastUpdate_X_a
  Display : Display
  Display1 : Display
  Manual Switch : ManualSwitch
  Manual Switch1 : ManualSwitch
  Scope4 : Scope
      settings: YMin=0  YMax=1  SaveName=ScopeData27
  Update with K(d) and update current state : Subsystem
  Update with K(k) and predict current state : Subsystem
  cov_nu : Constant  Value=Cov_nu
  cov_r : Constant  Value=Cov_r
  "ita " : Constant  Value=ita
  "rho " : Constant  Value=rho
  rho_c : Constant  Value=rho_c
  X_a_current : Outport
  P_post : Outport  Port=2
  X_a(k+1) : Outport  Port=3
  wires:
  Signal/1 -> Update with K(d) and update current state/6(signal), Update with K(k) and predict current state/4(signal)
  rho_c/1 -> Update with K(d) and update current state/7(rho_c), Update with K(k) and predict current state/5(rho_c)
  "ita "/1 -> Update with K(d) and update current state/4(ita), Update with K(k) and predict current state/6(ita)
  cov_r/1 -> Update with K(d) and update current state/5(Cov_r), Update with K(k) and predict current state/7(Cov_r)
  cov_nu/1 -> Update with K(d) and update current state/1(Cov_nu), Update with K(k) and predict current state/8(Cov_nu)
  Enable/1 -> Scope4/1
  Update with K(k) and predict current state/2(X_a_current) -> X_a_current/1
  del_t/1 -> Update with K(k) and predict current state/10(del_t)
  "q_nominal "/1 -> Create X from X_a/2(q_nominal(k)), Update with K(d) and update current state/2(q_nominal), Update with K(k) and predict current state/9(q_nominal)
  "rho "/1 -> Update with K(k) and predict current state/1(rho)
  Update with K(k) and predict current state/1(P_post) -> Manual Switch/1
  Create X from X_a/1(X(k)) -> Update with K(d) and update current state/3(X(k)), Update with K(k) and predict current state/2(X)
  X_a/1 -> Create X from X_a/1(X_a(k))
  P_pre/1 -> Update with K(k) and predict current state/3(P_pre), Update with K(d) and update current state/11(P_pre)
  Manual Switch/1 -> Display1/1, P_post/1
  Update with K(d) and update current state/2(P_present) -> Manual Switch/2
  Update with K(d) and update current state/1(X_a_present) -> Manual Switch1/2
  Update with K(k) and predict current state/3(X_a_k_1) -> Manual Switch1/1
  Manual Switch1/1 -> X_a(k+1)/1, Display/1, Data Store Write/1
  x_d/1 -> Update with K(d) and update current state/8(x_d)
  P_d/1 -> Update with K(d) and update current state/9(P_d)
  U_n_d/1 -> Update with K(d) and update current state/10(U_n_d)

== system EKF_04_2014/EKF/OOSM_KF ==
  "timestamp_cap " : Inport
  "meas_packet " : Inport  Port=2
  P_pre : Inport  Port=3
  X_a_\(k) : Inport  Port=4
  Constant : Constant  Value=0
  IC : InitialCondition  Value=0
  IC1 : InitialCondition  Value=0
  OOSM_KF : Subsystem
  OOSM_enable : Subsystem
  Scope : Scope
      settings: YMin=0  YMax=1  SaveName=ScopeData7
  U_n_d : Outport
  x_d : Outport  Port=2
  P_d : Outport  Port=3
  wires:
  "timestamp_cap "/1 -> OOSM_enable/1("timestamp_cap ")
  "meas_packet "/1 -> OOSM_enable/2(meas_packet)
  OOSM_enable/1(Trigger) -> IC/1
  Constant/1 -> OOSM_KF/1(del_t)
  OOSM_enable/2(reset_trigger) -> IC1/1
  IC/1 -> OOSM_KF/Enable, Scope/1
  IC1/1 -> OOSM_KF/2(reset_trigger)
  OOSM_enable/3("q_nominal ") -> OOSM_KF/3(q_nominal)
  OOSM_KF/1(U_n_d) -> U_n_d/1
  OOSM_KF/2(x_d) -> x_d/1
  OOSM_KF/3(P_d) -> P_d/1
  P_pre/1 -> OOSM_KF/4(P_pre(k))
  X_a_\(k)/1 -> OOSM_KF/5("x(k) ")

== system EKF_04_2014/EKF/Predictor ==
  X_a(K) : Inport
  P_previous(k) : Inport  Port=2
  trigger : Inport  Port=3
  X_a_present : Inport  Port=4
  Create Bus [State Vector,X_a] : Subsystem
  Create Bus [State Vector,X_a]1 : Subsystem
  Create Bus [State Vector,X_a]2 : Subsystem
  Create Bus [State Vector,X_a]3 : Subsystem
  Create State error covariance (P) : Subsystem
  Delay : Delay  DelayLength=1  InitialCondition=0
  Discrete-Time Integrator1 : DiscreteIntegrator  ExternalReset=rising  InitialConditionSource=external  InitialConditionSetting=State (most efficient)  SampleTime=-1
  Discrete-Time Integrator2 : DiscreteIntegrator  ExternalReset=rising  InitialConditionSource=external  InitialConditionSetting=State (most efficient)  SampleTime=-1
  Display : Display
  Dynamic Model (Differential equations)1 : Subsystem
  Dynamic Model (Differential equations)2 : Subsystem
  X_a(k+1) : Outport
  P_current(k+1) : Outport  Port=2
  X_present : Outport  Port=3
  wires:
  Create Bus [State Vector,X_a]1/1(X_bus) -> Create State error covariance (P)/1(X_a), Discrete-Time Integrator2/3
  Create State error covariance (P)/1(P_current) -> Display/1, P_current(k+1)/1
  Discrete-Time Integrator2/1 -> Create Bus [State Vector,X_a]/1(X)
  Dynamic Model (Differential equations)2/1(X_a_dot) -> Discrete-Time Integrator2/1
  P_previous(k)/1 -> Create State error covariance (P)/2(P_previous)
  trigger/1 -> Delay/1
  Create Bus [State Vector,X_a]/1(X_bus) -> X_a(k+1)/1
  X_a(K)/1 -> Dynamic Model (Differential equations)2/1(X_a(t)), Create Bus [State Vector,X_a]1/1(X)
  Delay/1 -> Discrete-Time Integrator2/2, Discrete-Time Integrator1/2
  Dynamic Model (Differential equations)1/1(X_a_dot) -> Discrete-Time Integrator1/1
  Discrete-Time Integrator1/1 -> Create Bus [State Vector,X_a]2/1(X)
  X_a_present/1 -> Dynamic Model (Differential equations)1/1(X_a(t)), Create Bus [State Vector,X_a]3/1(X)
  Create Bus [State Vector,X_a]2/1(X_bus) -> X_present/1
  Create Bus [State Vector,X_a]3/1(X_bus) -> Discrete-Time Integrator1/3

== system EKF_04_2014/Plant/Dynamic Model (Differential equations) ==
  X_a(t) : Inport
  Bus Creator : BusCreator
  Constant : Constant  Value=[0]
  "Orbital Dynamics " : Subsystem
  Quaternion Kinematics : Subsystem
  Rotational Dynamics : Subsystem
  Vector Concatenate : Concatenate
  n : Constant  Value=n
  omega : Selector  NumberOfDimensions=2  InputPortWidth=3  IndexOptions=Index vector (dialog),Index vector (dialog)  Indices=[5 6 7],1  OutputSizes=1,1
  p : Constant  Value=[p_x;p_y;p_z]
  parameter_gravitation : Constant  Value=parameter_gravitation
  q : Selector  NumberOfDimensions=2  InputPortWidth=3  IndexOptions=Index vector (dialog),Index vector (dialog)  Indices=[1 2 3 4],1  OutputSizes=1,1
  r : Selector  NumberOfDimensions=2  InputPortWidth=3  IndexOptions=Index vector (dialog),Index vector (dialog)  Indices=[8 9 10],1  OutputSizes=1,1
  r_dot : Selector  NumberOfDimensions=2  InputPortWidth=3  IndexOptions=Index vector (dialog),Index vector (dialog)  Indices=[11 12 13],1  OutputSizes=1,1
  X_a(t+1) : Outport
  wires:
  Constant/1 -> Vector Concatenate/2
  p/1 -> Rotational Dynamics/2(p)
  Vector Concatenate/1 -> Quaternion Kinematics/2(omega_rel)
  parameter_gravitation/1 -> "Orbital Dynamics "/2(Mu)
  n/1 -> "Orbital Dynamics "/3(n)
  "Orbital Dynamics "/1("r_ddot ") -> Bus Creator/4  "r_ddot"
  Quaternion Kinematics/1(q_dot) -> Bus Creator/1  "q_dot"
  Rotational Dynamics/1(omega_dot) -> Bus Creator/2  "omega_dot"
  X_a(t)/1 -> q/1, omega/1, r_dot/1, r/1
  q/1 -> Quaternion Kinematics/1(q)
  omega/1 -> Rotational Dynamics/1(omega), Vector Concatenate/1
  r/1 -> "Orbital Dynamics "/1(r)
  r_dot/1 -> "Orbital Dynamics "/4("r_dot "), Bus Creator/3
  Bus Creator/1 -> X_a(t+1)/1

== system EKF_04_2014/Plant/Initial Conditions (create bus) ==
  Bus Creator : BusCreator
  Bus Creator1 : BusCreator  Inputs=3
  Bus Creator2 : BusCreator  Inputs=3
  Bus Creator3 : BusCreator  Inputs=3
  Bus Creator4 : BusCreator
  Demux : Demux  Outputs=13
  Initial conditions (Dynamic Model) : FromFile  FileName=X_a_0_Model_02.mat  SampleTime=0
  "X_a(0) " : Outport
  wires:
  Initial conditions (Dynamic Model)/1 -> Demux/1
  Demux/1 -> Bus Creator/1  "q_1"
  Demux/2 -> Bus Creator/2  "q_2"
  Demux/3 -> Bus Creator/3  "q_3"
  Demux/4 -> Bus Creator/4  "q_0"
  Demux/5 -> Bus Creator1/1  "omega_x"
  Demux/6 -> Bus Creator1/2  "omega_y"
  Demux/7 -> Bus Creator1/3  "omega_z"
  Demux/8 -> Bus Creator2/1  "r_x"
  Demux/9 -> Bus Creator2/2  "r_y"
  Demux/10 -> Bus Creator2/3  "r_z"
  Demux/11 -> Bus Creator3/1  "r_x_dot"
  Demux/12 -> Bus Creator3/2  "r_y_dot"
  Demux/13 -> Bus Creator3/3  "r_z_dot"
  Bus Creator/1 -> Bus Creator4/1  "q"
  Bus Creator1/1 -> Bus Creator4/2  "omega"
  Bus Creator2/1 -> Bus Creator4/3  "r"
  Bus Creator3/1 -> Bus Creator4/4  "r_dot"
  Bus Creator4/1 -> "X_a(0) "/1  "X_a(0)"

== system EKF_04_2014/Plots and display/Create Measurements [Pose]1 ==
  q : Inport
  r : Inport  Port=2
  rho : Inport  Port=3
  ita : Inport  Port=4
  "rho_c " : Inport  Port=5
  "Create Measurements [Orientation] " : Subsystem
  Create Measurements [Position] : Subsystem
  Rate Transition : RateTransition
  Rate Transition1 : RateTransition
  Rate Transition2 : RateTransition
  r_c : Outport
  Mu : Outport  Port=2
  wires:
  q/1 -> "Create Measurements [Orientation] "/1(q), Create Measurements [Position]/2(q)
  r/1 -> Create Measurements [Position]/1(r)
  "Create Measurements [Orientation] "/1(Mu) -> Mu/1
  ita/1 -> Rate Transition1/1
  Create Measurements [Position]/1(r_c) -> r_c/1
  rho/1 -> Rate Transition2/1
  "rho_c "/1 -> Rate Transition/1
  Rate Transition/1 -> Create Measurements [Position]/4("rho_c ")
  Rate Transition1/1 -> "Create Measurements [Orientation] "/2("ita ")
  Rate Transition2/1 -> Create Measurements [Position]/3(rho)

== system EKF_04_2014/Plots and display/Create Measurements [Pose]2 ==
  q : Inport
  r : Inport  Port=2
  rho : Inport  Port=3
  ita : Inport  Port=4
  "rho_c " : Inport  Port=5
  "Create Measurements [Orientation] " : Subsystem
  Create Measurements [Position] : Subsystem
  Rate Transition : RateTransition
  Rate Transition1 : RateTransition
  Rate Transition2 : RateTransition
  r_c : Outport
  Mu : Outport  Port=2
  wires:
  Rate Transition2/1 -> Create Measurements [Position]/3(rho)
  Rate Transition1/1 -> "Create Measurements [Orientation] "/2("ita ")
  Rate Transition/1 -> Create Measurements [Position]/4("rho_c ")
  "rho_c "/1 -> Rate Transition/1
  rho/1 -> Rate Transition2/1
  Create Measurements [Position]/1(r_c) -> r_c/1
  ita/1 -> Rate Transition1/1
  "Create Measurements [Orientation] "/1(Mu) -> Mu/1
  r/1 -> Create Measurements [Position]/1(r)
  q/1 -> Create Measurements [Position]/2(q), "Create Measurements [Orientation] "/1(q)

== system EKF_04_2014/Create synthetic measurements [Pose]/Create Measurements [Orientation] /Quaternion norm ==
  q : Inport
  Demux3 : Demux
  Divide{,1..3} (4 alike) : Product  Inputs=*/
  Mux1 : Mux
  Norm(q) : Subsystem
  normalized_q : Outport
  wires:
  Demux3/3 -> Divide2/1
  Norm(q)/1(|q|) -> Divide3/2, Divide2/2, Divide1/2, Divide/2
  Demux3/1 -> Divide/1
  Divide3/1 -> Mux1/4
  Divide2/1 -> Mux1/3
  Mux1/1 -> normalized_q/1
  Demux3/2 -> Divide1/1
  q/1 -> Demux3/1, Norm(q)/1(q)
  Demux3/4 -> Divide3/1
  Divide/1 -> Mux1/1
  Divide1/1 -> Mux1/2
